simulink model "Solar_Seguidor"  (R2021b)
settings: Solver=ode1  StartTime=0.0  StopTime=inf  FixedStep=25e-6  RelTol=1e-3
PostLoadFcn:
  | %clc; clear all; close all;
  | %%%%%%%%%%%%%%%%%%%%%%%%%%%%%%%%%%%%%%%%%%%%%%%%
  | %%%%%%%%% Solar seguidor de rede %%%%%%%%%%
  | %%%%%%%%%%%%%%%%%%%%%%%%%%%%%%%%%%%%%%%%%%%%%%%%
  | %%%% Nominal Parameters %%%%
  | Pnom = 16e3;                                         % Potencia Nominal
  | Vnom_rms = 210;                                    % V linha rms
  | Vnom_peak = sqrt(2/3)*Vnom_rms;                     % V fase pico
  | FP_min = 1;                                       % Para suporte de reativo
  | Snom = Pnom/FP_min;                                 % Potencia aparente
  | Irms = Pnom/(sqrt(3)*Vnom_rms);                     % Ig rms
  | Inom_peak = Irms*sqrt(2);                           % Ig pico
  | Zbase = Vnom_peak/Inom_peak;                        % Impedancia Base
  | f = 60;                                             % Freq nominal
  | wnom = 2*pi*60;                                     % Freq Ang. nominal
  | m = 0.805;                                            % Indice mod nominal
  | Vdc = 2*(Vnom_peak/m);                              % Vcc
  | Vdc_2 = Vdc/2;                                      % Metade Vcc
  | Kconv = Zbase;                                      % Ganho conversor
  | %%%% Transformer %%%%
  | S_trafo = 250e3;                                      % transformer apparent power
  | Vrms_high = 400;                                   % transformer secondary voltage - Wye connection
  | Vrms_low = 210;                                   % transformer primary voltage - Delta connection
  | N = Vrms_high/Vrms_low;                             % transformation relationship
  | X_pu_trafo = 0.03;                                 % transformer p.u. reactance
  | Zb_trafo_high = ((Vrms_high)^2)/S_trafo;            % secondary base impedance
  | Zb_trafo = ((Vnom_rms)^2)/S_trafo;                  % primary base impedance
  | L_trafo = (X_pu_trafo*Zb_trafo)/wnom;               % primary inductance
  | %%%% LCL Filter Project %%%%
  | fsw = 105*60;%105*60;                                         % switching frequency
  | ripple = 0.05;                                       % current ripple
  | L1 = Vdc/(6*ripple*Inom_peak*fsw);                  % inductor L1
  |  RL1 = 0.005;                                        % L1 resistance
  |  Cbase = 1/(wnom*Kconv);                             % base capacitance
  |  Cf = 0.05*Cbase;                                    % filter capacitor
  | % Calculo do filtro
  | Sbase = 16e3;
  | %Sbase = 200e3*1.12;
  | V_LL = 210;
  | V_LG = 210/sqrt(3);
  | Vbase = V_LG*sqrt(2);
  | Ibase = (Sbase*sqrt(2))/(V_LG*3)*sqrt(3/2);
  | Zbase = (V_LL^2)/Sbase;
  | Rbase = Zbase;
  | Xbase = Zbase;
  | Lbase = Xbase/(2*pi*60);
  | Cbase = 1/(Xbase*2*pi*60);
  | w = 2*pi*60;
  | Q = 70;
  | Lf = 0.15*Lbase;
  | Cf = 0.05*Cbase;
  | fc = 1/(2*pi*sqrt(Lf*Cf));
  | R = (w*Lf)/Q;
  | Lf = L1;
  | R = RL1;
  | ka=0.2;                                             % attenuation factor
  | L2 = (sqrt(1/(ka^2))+1)/(Cf*((2*pi*fsw)^2));        % inductor L2
  | RL2 = 0.005;                                        % L2 resistance
  | w_res = sqrt((L1+L2+L_trafo)/(L1*L2*Cf));           % resonant angular frequency
  | f_res = w_res/(2*pi);                               % resonant frequency
  | ... (+31 lines)
InitFcn:
  | %clc; clear all; close all;
  | %%%%%%%%%%%%%%%%%%%%%%%%%%%%%%%%%%%%%%%%%%%%%%%%
  | %%%%%%%%% Solar seguidor de rede %%%%%%%%%%
  | %%%%%%%%%%%%%%%%%%%%%%%%%%%%%%%%%%%%%%%%%%%%%%%%
  | %%%% Nominal Parameters %%%%
  | Pnom = 16e3;                                         % Potencia Nominal
  | Vnom_rms = 210;                                    % V linha rms
  | Vnom_peak = sqrt(2/3)*Vnom_rms;                     % V fase pico
  | FP_min = 1;                                       % Para suporte de reativo
  | Snom = Pnom/FP_min;                                 % Potencia aparente
  | Irms = Pnom/(sqrt(3)*Vnom_rms);                     % Ig rms
  | Inom_peak = Irms*sqrt(2);                           % Ig pico
  | Zbase = Vnom_peak/Inom_peak;                        % Impedancia Base
  | f = 60;                                             % Freq nominal
  | wnom = 2*pi*60;                                     % Freq Ang. nominal
  | m = 0.805;                                            % Indice mod nominal
  | Vdc = 2*(Vnom_peak/m);                              % Vcc
  | Vdc_2 = Vdc/2;                                      % Metade Vcc
  | Kconv = Zbase;                                      % Ganho conversor
  | %%%% Transformer %%%%
  | S_trafo = 250e3;                                      % transformer apparent power
  | Vrms_high = 400;                                   % transformer secondary voltage - Wye connection
  | Vrms_low = 210;                                   % transformer primary voltage - Delta connection
  | N = Vrms_high/Vrms_low;                             % transformation relationship
  | X_pu_trafo = 0.03;                                 % transformer p.u. reactance
  | Zb_trafo_high = ((Vrms_high)^2)/S_trafo;            % secondary base impedance
  | Zb_trafo = ((Vnom_rms)^2)/S_trafo;                  % primary base impedance
  | L_trafo = (X_pu_trafo*Zb_trafo)/wnom;               % primary inductance
  | %%%% LCL Filter Project %%%%
  | fsw = 105*60;%105*60;                                         % switching frequency
  | ripple = 0.05;                                       % current ripple
  | L1 = Vdc/(6*ripple*Inom_peak*fsw);                  % inductor L1
  |  RL1 = 0.005;                                        % L1 resistance
  |  Cbase = 1/(wnom*Kconv);                             % base capacitance
  |  Cf = 0.05*Cbase;                                    % filter capacitor
  | % Calculo do filtro
  | Sbase = 16e3;
  | %Sbase = 200e3*1.12;
  | V_LL = 210;
  | V_LG = 210/sqrt(3);
  | Vbase = V_LG*sqrt(2);
  | Ibase = (Sbase*sqrt(2))/(V_LG*3)*sqrt(3/2);
  | Zbase = (V_LL^2)/Sbase;
  | Rbase = Zbase;
  | Xbase = Zbase;
  | Lbase = Xbase/(2*pi*60);
  | Cbase = 1/(Xbase*2*pi*60);
  | w = 2*pi*60;
  | Q = 70;
  | Lf = 0.15*Lbase;
  | Cf = 0.05*Cbase;
  | fc = 1/(2*pi*sqrt(Lf*Cf));
  | R = (w*Lf)/Q;
  | Lf = L1;
  | R = RL1;
  | ka=0.2;                                             % attenuation factor
  | L2 = (sqrt(1/(ka^2))+1)/(Cf*((2*pi*fsw)^2));        % inductor L2
  | RL2 = 0.005;                                        % L2 resistance
  | w_res = sqrt((L1+L2+L_trafo)/(L1*L2*Cf));           % resonant angular frequency
  | f_res = w_res/(2*pi);                               % resonant frequency
  | ... (+31 lines)
undefined symbols (not defined in the file): D1, Delta, DIN_2A_Ch00, DiscIntNeverNeededParam, eHS, I, Kp_dc, Left, parameter_set_id, ph, signal1, signal2, signal3, signal4, signal5, signal6, signal7, type, V
libraries: rtlab x11, spsCurrentMeasurementLib x4, spsabctodq0Lib x4, spsThreePhaseVIMeasurementLib x3, spsThreePhaseSeriesRLCBranchLib x3, spsPLL3phLib x3, spsTHDLib x3, artemis x2, spsOnDelayLib x2, spsSeriesRLCBranchLib x2, spsRMSLib x2, slpidlib x2
(part 2 of 2)

== system Solar_Seguidor/SM_mestre1/PV_system/Chopper ==
  Vdc : Inport
  Diode : spsDiodeLib/Diode  Ron=0.001  Lon=0  Vf=0.8  IC=0  UseSnubber=0  Rs=500  Cs=250e-9  Measurements=on
  Ideal Switch : spsIdealSwitchLib/Ideal Switch  Ron=0.001  Lon=0  IC=0  Rs=1e5  Cs=inf  Measurements=on
  Memory : Memory
  Relay1 : Relay  OnSwitchValue=1.1  OffSwitchValue=1.0
  Rtot_pu2 : Gain  Gain=1/Vdc  SaturateOnIntegerOverflow=on  OutDataTypeStr=Inherit: Same as input  ParamDataTypeStr=Inherit: Same as input
  Series RLC Branch1 : spsSeriesRLCBranchLib/Series RLC Branch  LConnTagsString=__new0  RConnTagsString=__new0  BranchType=R  Resistance=1.1*Vdc^2/Pnom  Inductance=1e-3  SetiL0=off  InitialCurrent=0  Capacitance=1e-6  Setx0=off  InitialVoltage=0  Measurements=None
  + : PMIOPort  Side=Left
  - : PMIOPort  Port=2  Side=Right
  wires:
  Vdc/1 -> Memory/1
  Relay1/1 -> Ideal Switch/1
  Memory/1 -> Rtot_pu2/1
  Rtot_pu2/1 -> Relay1/1
  connections:
  +/RConn1 -- Diode/RConn1 -- Ideal Switch/LConn1
  Ideal Switch/RConn1 -- Series RLC Branch1/LConn1 -- Diode/LConn1
  Series RLC Branch1/RConn1 -- -/RConn1

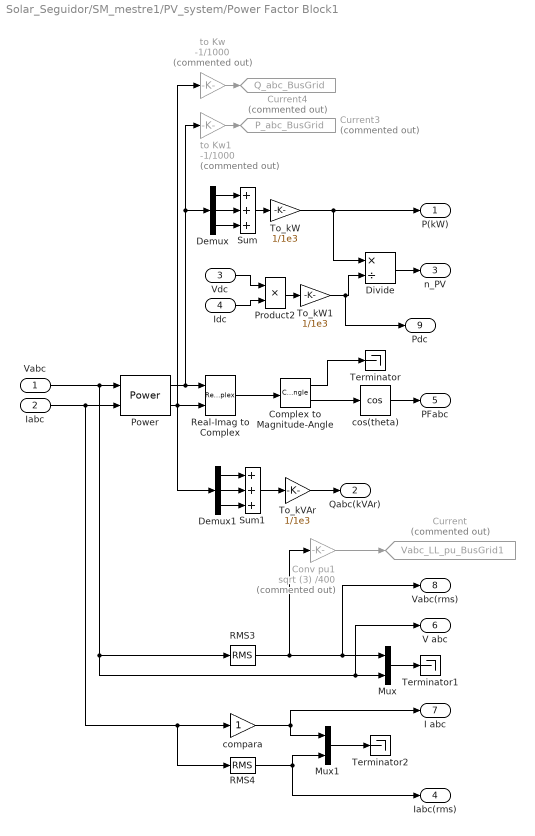
== system Solar_Seguidor/SM_mestre1/PV_system/Power Factor Block1 ==
  Vabc : Inport
  Iabc : Inport  Port=2
  Vdc : Inport  Port=3
  Idc : Inport  Port=4
  Complex to Magnitude-Angle : ComplexToMagnitudeAngle
  Conv pu1 : Gain  Commented=on  Gain=sqrt (3) /400  SaturateOnIntegerOverflow=on  OutDataTypeStr=Inherit: Same as input  ParamDataTypeStr=Inherit: Same as input
  Current : Goto  Commented=on  GotoTag=Vabc_LL_pu_BusGrid1  TagVisibility=global
  Current3 : Goto  Commented=on  GotoTag=P_abc_BusGrid  TagVisibility=global
  Current4 : Goto  Commented=on  GotoTag=Q_abc_BusGrid  TagVisibility=global
  Demux : Demux  Outputs=3
  Demux1 : Demux  Outputs=3
  Divide : Product  Inputs=*/
  Mux : Mux  Inputs=2
  Mux1 : Mux  Inputs=2
  Power : spsPowerLib/Power  Freq=Freq  Vinit=Vinit  Iinit=Iinit  Ts=Ts
      settings: SourceProductBaseCode=PS
  Product2 : Product
  RMS3 : spsRMSLib/RMS  TrueRMS=on  Freq=50  RMSInit=0  Ts=0
  RMS4 : spsRMSLib/RMS  TrueRMS=on  Freq=50  RMSInit=0  Ts=0
  Real-Imag to Complex : RealImagToComplex
  Sum : Sum  Inputs=+++
  Sum1 : Sum  Inputs=+++
  Terminator : Terminator
  Terminator1 : Terminator
  Terminator2 : Terminator
  To_kVAr : Gain  Gain=1/1e3
  To_kW : Gain  Gain=1/1e3
  To_kW1 : Gain  Gain=1/1e3
  compara : Gain  SaturateOnIntegerOverflow=on  OutDataTypeStr=Inherit: Same as input  ParamDataTypeStr=Inherit: Same as input
  cos(theta) : Trigonometry  Operator=cos
  to Kw : Gain  Commented=on  Gain=-1/1000
  to Kw1 : Gain  Commented=on  Gain=-1/1000
  P(kW) : Outport  VectorParamsAs1DForOutWhenUnconnected=off
  Qabc(kVAr) : Outport  Port=2  VectorParamsAs1DForOutWhenUnconnected=off
  n_PV : Outport  Port=3
  Iabc(rms) : Outport  Port=4  VectorParamsAs1DForOutWhenUnconnected=off
  "PFabc " : Outport  Port=5  VectorParamsAs1DForOutWhenUnconnected=off
  V abc : Outport  Port=6  VectorParamsAs1DForOutWhenUnconnected=off
  I abc : Outport  Port=7  VectorParamsAs1DForOutWhenUnconnected=off
  Vabc(rms) : Outport  Port=8  VectorParamsAs1DForOutWhenUnconnected=off
  Pdc : Outport  Port=9
  wires:
  Complex to Magnitude-Angle/2 -> cos(theta)/1
  Real-Imag to Complex/1 -> Complex to Magnitude-Angle/1
  cos(theta)/1 -> "PFabc "/1
  Complex to Magnitude-Angle/1 -> Terminator/1
  Iabc/1 -> RMS4/1, compara/1, Power/2
  RMS4/1 -> Iabc(rms)/1, Mux1/2
  Vabc/1 -> Power/1, V abc/1, Mux/2, RMS3/1
  RMS3/1 -> Conv pu1/1, Vabc(rms)/1, Mux/1
  Conv pu1/1 -> Current/1
  Power/1 -> to Kw1/1, Demux/1, Real-Imag to Complex/1
  to Kw/1 -> Current4/1
  to Kw1/1 -> Current3/1
  To_kVAr/1 -> Qabc(kVAr)/1
  Demux/1 -> Sum/1
  Demux/2 -> Sum/2
  Demux/3 -> Sum/3
  Sum/1 -> To_kW/1
  Demux1/3 -> Sum1/3
  Demux1/2 -> Sum1/2
  Demux1/1 -> Sum1/1
  Power/2 -> Demux1/1, to Kw/1, Real-Imag to Complex/2
  Sum1/1 -> To_kVAr/1
  compara/1 -> I abc/1, Mux1/1
  Mux/1 -> Terminator1/1
  Mux1/1 -> Terminator2/1
  Idc/1 -> Product2/2
  Vdc/1 -> Product2/1
  To_kW/1 -> P(kW)/1, Divide/1
  Divide/1 -> n_PV/1
  Product2/1 -> To_kW1/1
  To_kW1/1 -> Pdc/1, Divide/2

== system Solar_Seguidor/SM_mestre1/PV_system/Subsystem ==
  Current Measurement : spsCurrentMeasurementLib/Current Measurement  PhasorSimulation=off  OutputType=Complex  PSBequivalent=0
  Current Measurement1 : spsCurrentMeasurementLib/Current Measurement  PhasorSimulation=off  OutputType=Complex  PSBequivalent=0
  Current Measurement2 : spsCurrentMeasurementLib/Current Measurement  PhasorSimulation=off  OutputType=Complex  PSBequivalent=0
  Mux : Mux  Inputs=3
  a : PMIOPort  Side=Left
  Va : PMIOPort  Port=2  Side=Right
  b : PMIOPort  Port=3  Side=Left
  Vb : PMIOPort  Port=4  Side=Right
  c : PMIOPort  Port=5  Side=Left
  Vc : PMIOPort  Port=6  Side=Right
  Iabc : Outport
  wires:
  Current Measurement1/1 -> Mux/2
  Mux/1 -> Iabc/1
  Current Measurement/1 -> Mux/1
  Current Measurement2/1 -> Mux/3
  connections:
  Current Measurement2/RConn1 -- Vc/RConn1
  Current Measurement1/RConn1 -- Vb/RConn1
  Current Measurement/LConn1 -- a/RConn1
  Current Measurement2/LConn1 -- c/RConn1
  Current Measurement/RConn1 -- Va/RConn1
  b/RConn1 -- Current Measurement1/LConn1

== system Solar_Seguidor/SM_mestre1/PV_system/Subsystem1 ==
  Iabc : Inport
  In2 : Inport  Port=2
  Vdc : Inport  Port=3
  P_PV : Inport  Port=4
  Freq : Inport  Port=5
  Vabc : Inport  Port=6
  In7 : Inport  Port=7
  Vabc_rms : Inport  Port=8
  Bus Creator : BusCreator  Inputs=9
  Gain5 : Gain  Gain=1/(Ibase*1.27)
  Gain6 : Gain  Gain=1/(Ibase*1.15)
  THD : Subsystem
  Out1 : Outport
  wires:
  Iabc/1 -> THD/1(Iabc), Gain5/1
  Bus Creator/1 -> Out1/1
  THD/1(THD_I) -> Bus Creator/1  "THD_Ia"
  Gain6/1 -> Bus Creator/3  "Iabc_grid_pu"
  Gain5/1 -> Bus Creator/2  "Iabc_PV_pu"
  Freq/1 -> Bus Creator/6  "Freq"
  Vdc/1 -> Bus Creator/4  "Vdc"
  P_PV/1 -> Bus Creator/5  "P_PV"
  In2/1 -> Gain6/1
  Vabc/1 -> Bus Creator/7  "Vabc_grid"
  In7/1 -> Bus Creator/8  "Iabc_rms"
  Vabc_rms/1 -> Bus Creator/9  "Vabc_rms"

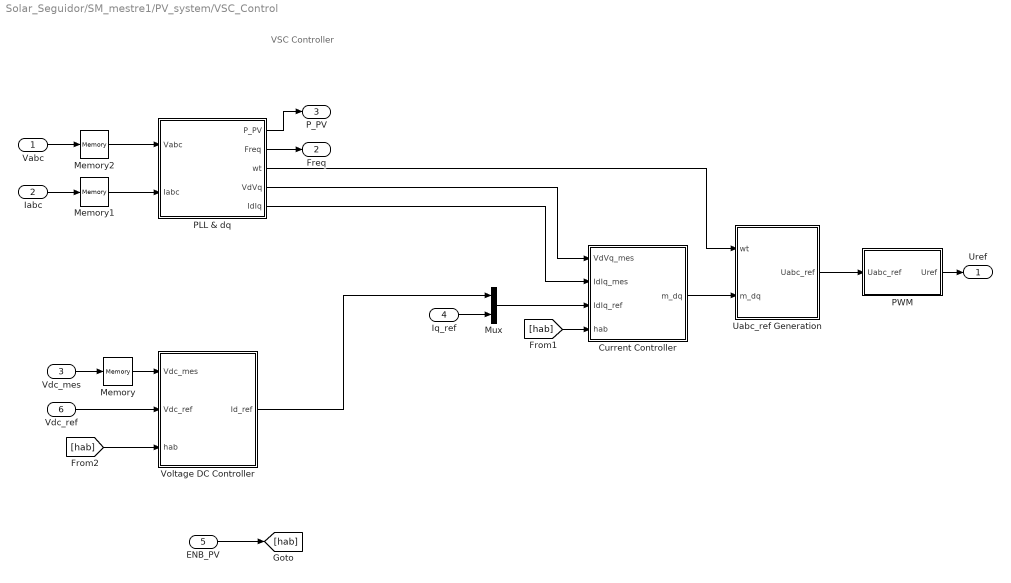
== system Solar_Seguidor/SM_mestre1/PV_system/VSC_Control ==
  note: VSC Controller
  Vabc : Inport  PortDimensions=3
  Iabc : Inport  Port=2  PortDimensions=3
  Vdc_mes : Inport  Port=3
  Iq_ref : Inport  Port=4
  ENB_PV : Inport  Port=5
  Vdc_ref : Inport  Port=6
  Current Controller : Subsystem
  Memory : Memory
  Memory1 : Memory
  Memory2 : Memory
  Mux : Mux  Inputs=2
  PLL & dq : Subsystem
  PWM : Subsystem
  "Uabc_ref Generation " : Subsystem
  Voltage DC Controller : Subsystem
  Uref : Outport  VectorParamsAs1DForOutWhenUnconnected=off
  Freq : Outport  Port=2
  P_PV : Outport  Port=3
  wires:
  [hab] -> Current Controller/4(hab)
  "Uabc_ref Generation "/1(Uabc_ref) -> PWM/1(Uabc_ref)
  PLL & dq/2(Freq) -> Freq/1
  PLL & dq/3(wt) -> "Uabc_ref Generation "/1(wt)
  PLL & dq/5(IdIq) -> Current Controller/2(IdIq_mes)
  Mux/1 -> Current Controller/3(IdIq_ref)
  PLL & dq/4(VdVq) -> Current Controller/1(VdVq_mes)
  Iq_ref/1 -> Mux/2
  Current Controller/1(m_dq) -> "Uabc_ref Generation "/2(m_dq)
  ENB_PV/1 -> [hab]
  [hab] -> Voltage DC Controller/3(hab)
  Vdc_mes/1 -> Memory/1
  PLL & dq/1(P_PV) -> P_PV/1
  Memory/1 -> Voltage DC Controller/1(Vdc_mes)
  Iabc/1 -> Memory1/1
  Memory1/1 -> PLL & dq/2(Iabc)
  Vabc/1 -> Memory2/1
  Memory2/1 -> PLL & dq/1(Vabc)
  Voltage DC Controller/1(Id_ref) -> Mux/1
  Vdc_ref/1 -> Voltage DC Controller/2(Vdc_ref)
  PWM/1(Uref) -> Uref/1

== system Solar_Seguidor/SM_mestre1/PV_system/Subsystem1/THD ==
  Iabc : Inport
  Demux : Demux  Outputs=3
  Gain1 : Gain  Gain=100
  Gain2 : Gain  Gain=100
  Gain3 : Gain  Gain=100
  Mux : Mux  Inputs=3
  Saturation : Saturate  UpperLimit=7
  Saturation1 : Saturate  UpperLimit=7
  Saturation2 : Saturate  UpperLimit=7
  THD : spsTHDLib/THD  Freq=60  Ts=Ts
      settings: SourceProductBaseCode=PS
  THD1 : spsTHDLib/THD  Freq=60  Ts=Ts
      settings: SourceProductBaseCode=PS
  THD2 : spsTHDLib/THD  Freq=60  Ts=Ts
      settings: SourceProductBaseCode=PS
  THD_I : Outport
  wires:
  Demux/1 -> THD/1
  Saturation2/1 -> Mux/3
  Saturation/1 -> Mux/1
  THD/1 -> Gain1/1
  Saturation1/1 -> Mux/2
  Demux/3 -> THD2/1
  THD1/1 -> Gain2/1
  Gain2/1 -> Saturation1/1
  Gain3/1 -> Saturation2/1
  THD2/1 -> Gain3/1
  Demux/2 -> THD1/1
  Gain1/1 -> Saturation/1
  Iabc/1 -> Demux/1
  Mux/1 -> THD_I/1

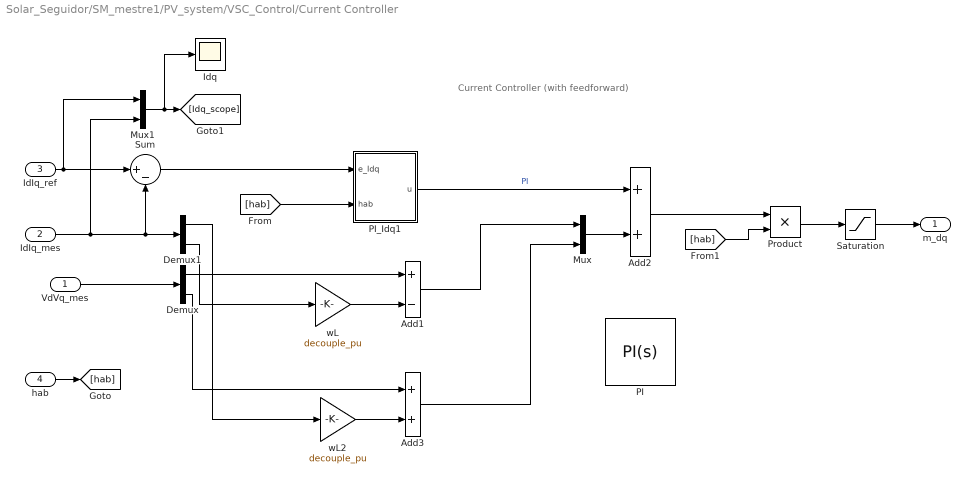
== system Solar_Seguidor/SM_mestre1/PV_system/VSC_Control/Current Controller ==
  note: Current Controller (with feedforward)
  VdVq_mes : Inport  PortDimensions=2
  IdIq_mes : Inport  Port=2  PortDimensions=2
  IdIq_ref : Inport  Port=3  PortDimensions=2
  hab : Inport  Port=4
  Add1 : Sum  Inputs=+-
  Add2 : Sum
  Add3 : Sum
  Demux : Demux  Outputs=2
  Demux1 : Demux  Outputs=2
  Idq : Scope
  Mux : Mux  Inputs=2
  Mux1 : Mux  Inputs=2
  PI : slpidlib/PID Controller  Controller=PI  Form=Parallel  TimeDomain=Continuous-time  UseExternalTs=off  SampleTime=Ts  IntegratorMethod=Forward Euler  FilterMethod=Forward Euler  ControllerParametersSource=internal  P=kp_current_pu  I=ki_current_pu  D=0  UseFilter=on  N=100  TunerSelectOption=Transfer Function Based (PID Tuner App)  InitialConditionSource=internal  InitialConditionForIntegrator=0  InitialConditionForFilter=0  DifferentiatorICPrevScaledInput=0  ExternalReset=rising  TrackingMode=off  Kt=1  LimitOutput=off  SatLimitsSource=internal  UpperSaturationLimit=2  LowerSaturationLimit=-2  LinearizeAsGain=off  AntiWindupMode=none  Kb=1  POutMin=[]  POutMax=[]  IOutMin=[]  IOutMax=[]  DOutMin=[]  DOutMax=[]  NOutMin=[]  NOutMax=[]  SumOutMin=[]  SumOutMax=[]  SaturationOutMin=[]  SaturationOutMax=[]  PParamMin=[]  PParamMax=[]  IParamMin=[]  IParamMax=[]  DParamMin=[]  DParamMax=[]  NParamMin=[]  NParamMax=[]  KbParamMin=[]  KbParamMax=[]  KtParamMin=[]  KtParamMax=[]  KbOutMin=[]  KbOutMax=[]  KtOutMin=[]  KtOutMax=[]  IntegratorOutMin=[]  IntegratorOutMax=[]  FilterOutMin=[]  FilterOutMax=[]  SumI1OutMin=[]  SumI1OutMax=[]  SumI2OutMin=[]  SumI2OutMax=[]  SumI3OutMin=[]  SumI3OutMax=[]  SumI4OutMin=[]  SumI4OutMax=[]  SumDOutMin=[]  SumDOutMax=[]  DifferentiatorOutMin=[]  DifferentiatorOutMax=[]  FilterDiffOutCoefMin=[]  FilterDiffOutCoefMax=[]  ReciprocalOutMin=[]  ReciprocalOutMax=[]  SumDenOutMin=[]  SumDenOutMax=[]  SumNumOutMin=[]  SumNumOutMax=[]  DivideOutMin=[]  DivideOutMax=[]  UdiffTsProdOutMin=[]  UdiffTsProdOutMax=[]  NTsProdOutMin=[]  NTsProdOutMax=[]  UintegralTsProdOutMin=[]  UintegralTsProdOutMax=[]  UngainTsProdOutMin=[]  UngainTsProdOutMax=[]  FilterDenConstantOutDataTypeStr=Inherit: Inherit via back propagation  FilterDenConstantOutMin=[]  FilterDenConstantOutMax=[]  PCopyOutDataTypeStr=Inherit: Inherit via back propagation  PCopyOutMin=[]  PCopyOutMax=[]  NCopyOutDataTypeStr=Inherit: Inherit via back propagation  NCopyOutMin=[]  NCopyOutMax=[]  IntegratorContinuousStateAttributes=''  IntegratorStateMustResolveToSignalObject=off  IntegratorRTWStateStorageClass=Auto  FilterContinuousStateAttributes=''  FilterStateMustResolveToSignalObject=off  FilterRTWStateStorageClass=Auto  ParallelPVariant=InternalParameters  IdealPVariant=Disabled  IVariant=InternalParameters  DVariant=Disabled  IntegratorVariant=Continuous  SatVariant=Disabled  AWVariant=Passthrough  PCopyVariant=Disabled  TRVariant=Disabled  FdbkBlocksVariant=Forward  IdealPFdbkVariant=Disabled  SatFdbkVariant=Disabled  DerivativeFilterVariant=Disabled  NVariant=Disabled  NCopyVariant=Disabled_SignalSpec  FilterICVariant=Disabled  IntegratorICVariant=InternalICs  ExternalResetVariant=ExternalReset  TRSumVariant=Passthrough  SumFdbkVariant=Disabled  SumVariant=Sum_PI  TsampFilterVariant=InternalTs  TsampNgainVariant=Passthrough  TsampIntegralVariant=Passthrough  ExternalSaturationOutDataTypeStr=Inherit: Same as second input
  PI_Idq1 : Subsystem
  Product : Product
  Saturation : Saturate  UpperLimit=10  LowerLimit=-10
  Sum : Sum  Inputs=|+-
  wL : Gain  Gain=decouple_pu  SaturateOnIntegerOverflow=on  OutDataTypeStr=Inherit: Same as input  ParamDataTypeStr=Inherit: Same as input
  wL2 : Gain  Gain=decouple_pu  SaturateOnIntegerOverflow=on  OutDataTypeStr=Inherit: Same as input  ParamDataTypeStr=Inherit: Same as input
  m_dq : Outport  VectorParamsAs1DForOutWhenUnconnected=off
  wires:
  wL/1 -> Add1/2
  Mux/1 -> Add2/2
  PI_Idq1/1(u) -> Add2/1  "PI"
  Sum/1 -> PI_Idq1/1(e_Idq)
  Saturation/1 -> m_dq/1
  VdVq_mes/1 -> Demux/1
  Demux/1 -> Add1/1
  Demux1/1 -> wL2/1
  Demux1/2 -> wL/1
  wL2/1 -> Add3/2
  Add1/1 -> Mux/1
  Demux/2 -> Add3/1
  Add3/1 -> Mux/2
  Add2/1 -> Product/1
  Product/1 -> Saturation/1
  hab/1 -> [hab]
  [hab] -> PI_Idq1/2(hab)
  [hab] -> Product/2
  Mux1/1 -> Idq/1, [Idq_scope]
  IdIq_ref/1 -> Mux1/1, Sum/1
  IdIq_mes/1 -> Mux1/2, Sum/2, Demux1/1

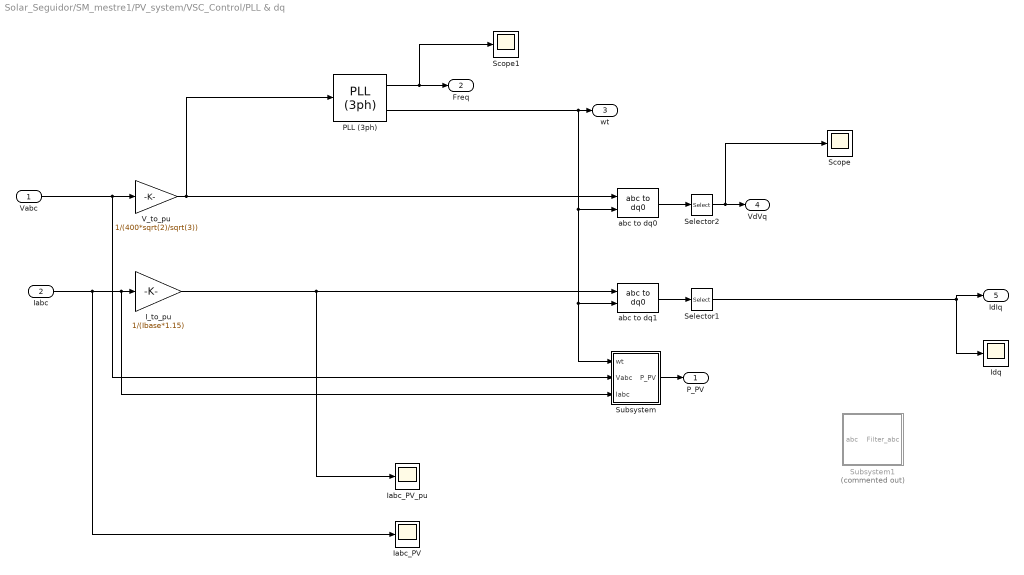
== system Solar_Seguidor/SM_mestre1/PV_system/VSC_Control/PLL & dq ==
  Vabc : Inport
  Iabc : Inport  Port=2
  I_to_pu : Gain  Gain=1/(Ibase*1.15)  SaturateOnIntegerOverflow=on  OutDataTypeStr=Inherit: Same as input  ParamDataTypeStr=Inherit: Same as input
  Iabc_PV : Scope
  Iabc_PV_pu : Scope
  Idq : Scope
  PLL (3ph) : spsPLL3phLib/PLL (3ph)  Fmin=45  Par_Init="[-0.57  60]"  ParK=[180, 3200, 1]  TcD=Ts_Control  MaxRateChangeFreq=12  FilterCutOffFreq=25  Ts=Ts_Control  AGC=on
  Scope : Scope
  Scope1 : Scope
  Selector1 : Selector  InputPortWidth=3  IndexOptions=Index vector (dialog)  Indices=[1 2]  OutputSizes=1
  Selector2 : Selector  InputPortWidth=3  IndexOptions=Index vector (dialog)  Indices=[1 2]  OutputSizes=1
  Subsystem : Subsystem
  Subsystem1 : Subsystem  Commented=on
  V_to_pu : Gain  Gain=1/(400*sqrt(2)/sqrt(3))  SaturateOnIntegerOverflow=on  OutDataTypeStr=Inherit: Same as input  ParamDataTypeStr=Inherit: Same as input
  abc to dq0 : spsabctodq0Lib/abc to dq0  Alignment=90 degrees behind phase A axis
  abc to dq1 : spsabctodq0Lib/abc to dq0  Alignment=90 degrees behind phase A axis
  P_PV : Outport
  Freq : Outport  Port=2
  wt : Outport  Port=3  VectorParamsAs1DForOutWhenUnconnected=off
  VdVq : Outport  Port=4  VectorParamsAs1DForOutWhenUnconnected=off
  IdIq : Outport  Port=5  VectorParamsAs1DForOutWhenUnconnected=off
  wires:
  Iabc/1 -> Iabc_PV/1, Subsystem/3(Iabc), I_to_pu/1
  I_to_pu/1 -> Iabc_PV_pu/1, abc to dq1/1
  V_to_pu/1 -> abc to dq0/1, PLL (3ph)/1
  abc to dq1/1 -> Selector1/1
  Vabc/1 -> Subsystem/2(Vabc), V_to_pu/1
  abc to dq0/1 -> Selector2/1
  PLL (3ph)/1 -> Scope1/1, Freq/1
  Selector2/1 -> Scope/1, VdVq/1
  Subsystem/1(P_PV) -> P_PV/1
  PLL (3ph)/2 -> Subsystem/1(wt), abc to dq1/2, abc to dq0/2, wt/1
  Selector1/1 -> IdIq/1, Idq/1

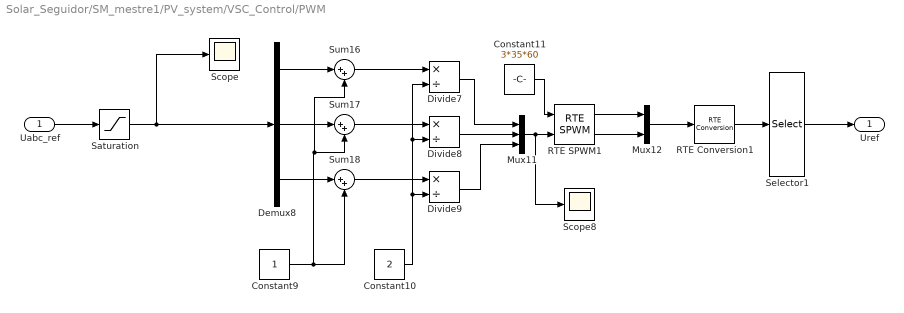
== system Solar_Seguidor/SM_mestre1/PV_system/VSC_Control/PWM ==
  Uabc_ref : Inport
  Constant10 : Constant  Value=2
  Constant11 : Constant  Value=3*35*60
  Constant9 : Constant
  Demux8 : Demux  Outputs=3
  Divide7 : Product  Inputs=*/
  Divide8 : Product  Inputs=*/
  Divide9 : Product  Inputs=*/
  Mux11 : Mux  Inputs=3
  Mux12 : Mux  Inputs=2
  RTE Conversion1 : rteventslib/Signal Attributes/RTE Conversion  inputdatatype=RTE Boolean  outputdatatype=Double  compensation=Enabled  nbMaxEvents=4  sampleTime=Ts
  RTE SPWM1 : rteventslib/Sources/RTE SPWM  NumberPhases=3-ph  CenterAlignmentMode=On  MaxFreq=inf  MinFreq=0  EnablingPort=off  ComplementaryMode=on  SpaceVector=off  RiseTimeDelay=0  MaxEvents=4  SampleTime=Ts
  Saturation : Saturate  UpperLimit=2  LowerLimit=-2
  Scope : Scope
  Scope8 : Scope
  Selector1 : Selector  InputPortWidth=6  IndexOptions=Index vector (dialog)  Indices=[1 4 2 5 3 6]  OutputSizes=1
  Sum16 : Sum  Inputs=|++
  Sum17 : Sum  Inputs=|++
  Sum18 : Sum  Inputs=|++
  Uref : Outport  VectorParamsAs1DForOutWhenUnconnected=off
  wires:
  RTE Conversion1/1 -> Selector1/1
  Mux12/1 -> RTE Conversion1/1
  Demux8/3 -> Sum18/1
  Demux8/1 -> Sum16/1
  Divide7/1 -> Mux11/1
  Mux11/1 -> Scope8/1, RTE SPWM1/2
  Sum18/1 -> Divide9/1
  Divide8/1 -> Mux11/2
  Demux8/2 -> Sum17/1
  Uabc_ref/1 -> Saturation/1
  RTE SPWM1/2 -> Mux12/2
  Divide9/1 -> Mux11/3
  Sum17/1 -> Divide8/1
  Constant10/1 -> Divide7/2, Divide8/2, Divide9/2
  Sum16/1 -> Divide7/1
  Constant11/1 -> RTE SPWM1/1
  Selector1/1 -> Uref/1
  Constant9/1 -> Sum16/2, Sum17/2, Sum18/2
  RTE SPWM1/1 -> Mux12/1
  Saturation/1 -> Scope/1, Demux8/1

== system Solar_Seguidor/SM_mestre1/PV_system/VSC_Control/Uabc_ref Generation  ==
  note: Uabc_ref Generation
  wt : Inport
  m_dq : Inport  Port=2
  Constant5 : Constant  Value=0
  Mux : Mux  Inputs=2
  Scope : Scope
  dq0 to abc : spsdq0toabcLib/dq0 to abc  Alignment=90 degrees behind phase A axis
  Uabc_ref : Outport  VectorParamsAs1DForOutWhenUnconnected=off
  wires:
  Mux/1 -> dq0 to abc/1
  Constant5/1 -> Mux/2
  wt/1 -> dq0 to abc/2
  dq0 to abc/1 -> Uabc_ref/1
  m_dq/1 -> Scope/1, Mux/1

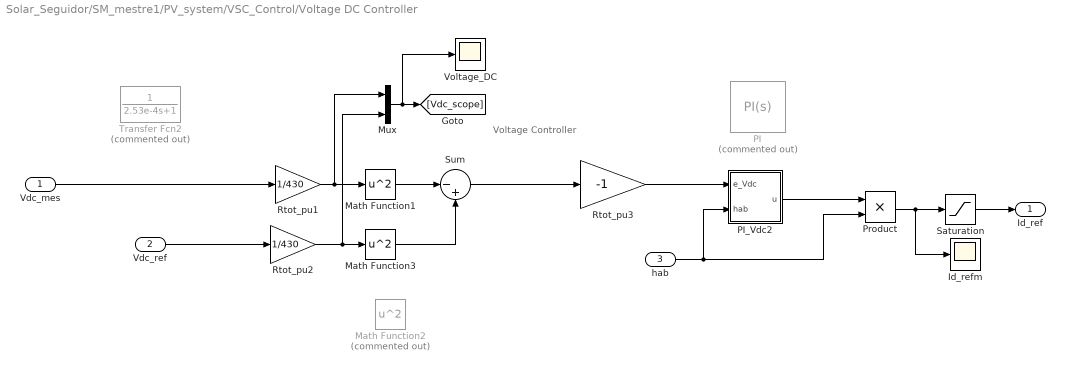
== system Solar_Seguidor/SM_mestre1/PV_system/VSC_Control/Voltage DC Controller ==
  note: Voltage Controller
  Vdc_mes : Inport  PortDimensions=1
  Vdc_ref : Inport  Port=2  PortDimensions=1
  hab : Inport  Port=3
  Id_refm : Scope
  Math Function1 : Math  Operator=square  SaturateOnIntegerOverflow=on
  Math Function2 : Math  Commented=on  Operator=square  SaturateOnIntegerOverflow=on
  Math Function3 : Math  Operator=square  SaturateOnIntegerOverflow=on
  Mux : Mux  Inputs=2
  PI : slpidlib/PID Controller  Commented=on  Controller=PI  Form=Parallel  TimeDomain=Continuous-time  UseExternalTs=off  SampleTime=Ts  IntegratorMethod=Trapezoidal  FilterMethod=Forward Euler  ControllerParametersSource=internal  P=Kp_dc  I=ki_dc_pu  D=0  UseFilter=on  N=100  TunerSelectOption=Transfer Function Based (PID Tuner App)  InitialConditionSource=internal  InitialConditionForIntegrator=0  InitialConditionForFilter=0  DifferentiatorICPrevScaledInput=0  ExternalReset=rising  TrackingMode=off  Kt=1  LimitOutput=on  SatLimitsSource=internal  UpperSaturationLimit=1.4  LowerSaturationLimit=-2  LinearizeAsGain=off  AntiWindupMode=clamping  Kb=1  POutMin=[]  POutMax=[]  IOutMin=[]  IOutMax=[]  DOutMin=[]  DOutMax=[]  NOutMin=[]  NOutMax=[]  SumOutMin=[]  SumOutMax=[]  SaturationOutMin=[]  SaturationOutMax=[]  PParamMin=[]  PParamMax=[]  IParamMin=[]  IParamMax=[]  DParamMin=[]  DParamMax=[]  NParamMin=[]  NParamMax=[]  KbParamMin=[]  KbParamMax=[]  KtParamMin=[]  KtParamMax=[]  KbOutMin=[]  KbOutMax=[]  KtOutMin=[]  KtOutMax=[]  IntegratorOutMin=[]  IntegratorOutMax=[]  FilterOutMin=[]  FilterOutMax=[]  SumI1OutMin=[]  SumI1OutMax=[]  SumI2OutMin=[]  SumI2OutMax=[]  SumI3OutMin=[]  SumI3OutMax=[]  SumI4OutMin=[]  SumI4OutMax=[]  SumDOutMin=[]  SumDOutMax=[]  DifferentiatorOutMin=[]  DifferentiatorOutMax=[]  FilterDiffOutCoefMin=[]  FilterDiffOutCoefMax=[]  ReciprocalOutMin=[]  ReciprocalOutMax=[]  SumDenOutMin=[]  SumDenOutMax=[]  SumNumOutMin=[]  SumNumOutMax=[]  DivideOutMin=[]  DivideOutMax=[]  UdiffTsProdOutMin=[]  UdiffTsProdOutMax=[]  NTsProdOutMin=[]  NTsProdOutMax=[]  UintegralTsProdOutMin=[]  UintegralTsProdOutMax=[]  UngainTsProdOutMin=[]  UngainTsProdOutMax=[]  FilterDenConstantOutDataTypeStr=Inherit: Inherit via back propagation  FilterDenConstantOutMin=[]  FilterDenConstantOutMax=[]  PCopyOutDataTypeStr=Inherit: Inherit via back propagation  PCopyOutMin=[]  PCopyOutMax=[]  NCopyOutDataTypeStr=Inherit: Inherit via back propagation  NCopyOutMin=[]  NCopyOutMax=[]  IntegratorContinuousStateAttributes=''  IntegratorStateMustResolveToSignalObject=off  IntegratorRTWStateStorageClass=Auto  FilterContinuousStateAttributes=''  FilterStateMustResolveToSignalObject=off  FilterRTWStateStorageClass=Auto  ParallelPVariant=InternalParameters  IdealPVariant=Disabled  IVariant=InternalParameters  DVariant=Disabled  IntegratorVariant=Continuous  SatVariant=Enabled  AWVariant=ContClampingParallel  PCopyVariant=Disabled  TRVariant=Disabled  FdbkBlocksVariant=Forward  IdealPFdbkVariant=Disabled  SatFdbkVariant=Disabled  DerivativeFilterVariant=Disabled  NVariant=Disabled  NCopyVariant=Disabled_SignalSpec  FilterICVariant=Disabled  IntegratorICVariant=InternalICs  ExternalResetVariant=ExternalReset  TRSumVariant=Passthrough  SumFdbkVariant=Disabled  SumVariant=Sum_PI  TsampFilterVariant=InternalTs  TsampNgainVariant=Passthrough  TsampIntegralVariant=Passthrough  ExternalSaturationOutDataTypeStr=Inherit: Same as second input
  PI_Vdc2 : Subsystem
  Product : Product
  Rtot_pu1 : Gain  Gain=1/430  SaturateOnIntegerOverflow=on  OutDataTypeStr=Inherit: Same as input  ParamDataTypeStr=Inherit: Same as input
  Rtot_pu2 : Gain  Gain=1/430  SaturateOnIntegerOverflow=on  OutDataTypeStr=Inherit: Same as input  ParamDataTypeStr=Inherit: Same as input
  Rtot_pu3 : Gain  Gain=-1  SaturateOnIntegerOverflow=on  OutDataTypeStr=Inherit: Same as input  ParamDataTypeStr=Inherit: Same as input
  Saturation : Saturate  UpperLimit=1.1  LowerLimit=0
  Sum : Sum  Inputs=|-+
  Transfer Fcn2 : TransferFcn  Commented=on  Denominator=[2.53e-4 1]
  Voltage_DC : Scope
  Id_ref : Outport  SampleTime=Ts  InitialOutput=0  VectorParamsAs1DForOutWhenUnconnected=off
  wires:
  Rtot_pu3/1 -> PI_Vdc2/1(e_Vdc)
  Vdc_ref/1 -> Rtot_pu2/1
  Sum/1 -> Rtot_pu3/1
  hab/1 -> Product/2, PI_Vdc2/2(hab)
  Mux/1 -> Voltage_DC/1, [Vdc_scope]
  Rtot_pu1/1 -> Mux/1, Math Function1/1
  Rtot_pu2/1 -> Mux/2, Math Function3/1
  Math Function1/1 -> Sum/1
  Math Function3/1 -> Sum/2
  Vdc_mes/1 -> Rtot_pu1/1
  Saturation/1 -> Id_ref/1
  PI_Vdc2/1(u) -> Product/1
  Product/1 -> Id_refm/1, Saturation/1

== system Solar_Seguidor/SM_mestre1/PV_system/VSC_Control/Current Controller/PI_Idq1 ==
  e_Idq : Inport
  hab : Inport  Port=2
  Discrete-Time Integrator : DiscreteIntegrator  SampleTime=-1  ICPrevOutput=DiscIntNeverNeededParam  ICPrevScaledInput=DiscIntNeverNeededParam
  Gain1 : Gain  Gain=kp_current_pu
  Gain2 : Gain  Gain=ki_current_pu
  Product : Product
  Sum1 : Sum
  u : Outport
  wires:
  hab/1 -> Product/2
  e_Idq/1 -> Product/1
  Discrete-Time Integrator/1 -> Sum1/2
  Sum1/1 -> u/1
  Gain1/1 -> Sum1/1
  Product/1 -> Gain2/1, Gain1/1
  Gain2/1 -> Discrete-Time Integrator/1

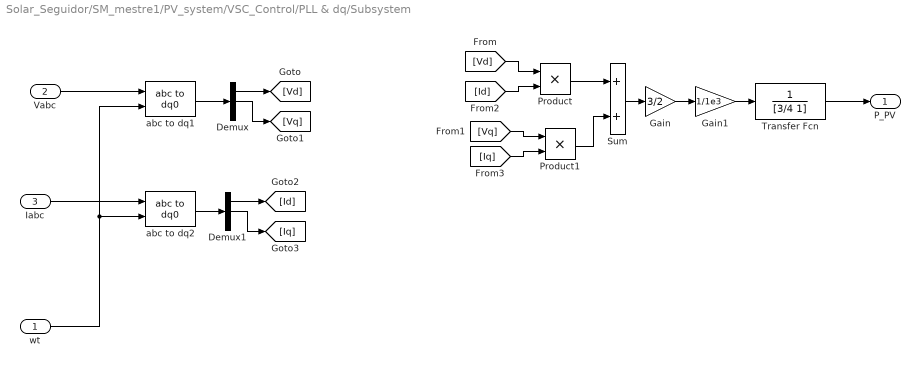
== system Solar_Seguidor/SM_mestre1/PV_system/VSC_Control/PLL & dq/Subsystem ==
  wt : Inport
  Vabc : Inport  Port=2
  Iabc : Inport  Port=3
  Demux : Demux  Outputs=3
  Demux1 : Demux  Outputs=3
  Gain : Gain  Gain=3/2
  Gain1 : Gain  Gain=1/1e3
  Product : Product
  Product1 : Product
  Sum : Sum
  Transfer Fcn : TransferFcn  Denominator=[3/4 1]
  abc to dq1 : spsabctodq0Lib/abc to dq0  Alignment=90 degrees behind phase A axis
  abc to dq2 : spsabctodq0Lib/abc to dq0  Alignment=90 degrees behind phase A axis
  P_PV : Outport
  wires:
  [Id] -> Product/2
  Product/1 -> Sum/1
  Gain1/1 -> Transfer Fcn/1
  [Vd] -> Product/1
  Gain/1 -> Gain1/1
  [Iq] -> Product1/2
  Sum/1 -> Gain/1
  Product1/1 -> Sum/2
  Transfer Fcn/1 -> P_PV/1
  [Vq] -> Product1/1
  Vabc/1 -> abc to dq1/1
  wt/1 -> abc to dq2/2, abc to dq1/2
  Iabc/1 -> abc to dq2/1
  abc to dq1/1 -> Demux/1
  Demux/1 -> [Vd]
  Demux/2 -> [Vq]
  Demux1/2 -> [Iq]
  Demux1/1 -> [Id]
  abc to dq2/1 -> Demux1/1

== system Solar_Seguidor/SM_mestre1/PV_system/VSC_Control/PLL & dq/Subsystem1 ==
  abc : Inport
  Demux : Demux  Outputs=2
  Mux1 : Mux  Inputs=2
  Transfer Fcn1 : TransferFcn  Denominator=[2.53e-4 1]
  Transfer Fcn4 : TransferFcn  Denominator=[2.53e-4 1]
  Filter_abc : Outport
  wires:
  Demux/1 -> Transfer Fcn4/1
  Transfer Fcn4/1 -> Mux1/1
  Transfer Fcn1/1 -> Mux1/2
  Mux1/1 -> Filter_abc/1
  Demux/2 -> Transfer Fcn1/1
  abc/1 -> Demux/1

== system Solar_Seguidor/SM_mestre1/PV_system/VSC_Control/Voltage DC Controller/PI_Vdc2 ==
  e_Vdc : Inport
  hab : Inport  Port=2
  Discrete-Time Integrator : DiscreteIntegrator  SampleTime=-1  ICPrevOutput=DiscIntNeverNeededParam  ICPrevScaledInput=DiscIntNeverNeededParam
  Gain1 : Gain  Gain=kp_dc_pu
  Gain2 : Gain  Gain=ki_dc_pu
  Product : Product
  Sum1 : Sum
  u : Outport
  wires:
  Gain2/1 -> Discrete-Time Integrator/1
  Product/1 -> Gain1/1, Gain2/1
  Gain1/1 -> Sum1/1
  Sum1/1 -> u/1
  Discrete-Time Integrator/1 -> Sum1/2
  e_Vdc/1 -> Product/1
  hab/1 -> Product/2
